simulink model "Track_model_wtihtesting_datacooling"  (R2024a)
settings: Solver=FixedStepAuto  StartTime=0.0  StopTime=1200  FixedStep=0.01  MaxStep=1e-2  MinStep=1e-5  RelTol=1e-3  AbsTol=1e-11
PreLoadFcn:
  | Straight1_Track = [75	3.446	29.063	1.834	47.653	8.247	3.373	13.154	57.193	39.54	5.916	3.204	2.701	2.747	90.673	4.72	3.366	94.658	23.788	1	40.161	15.969	17.891	3.717	36.358	76.419	54.208	36.993	4.775	55.007	1.783	4.349
  | ];
  | Curved_Track = [13.325	13.688	13.825	14.949	16.182	52.505	18.752	19.67	17.192	18.934	14.945	16.948	14.677	9.353	16.047	6.011	19.463	14.821	17.716	9.886	20.496	17.101	19.463	24.351	37.401	18.473	21.711	5.558	59.024	6.989	13.452	41.008
  | ];
  | Radius1 = [12	16.8	16.75	13.5	18.6	22.46	17.818	17.73	14	25.6	16.44	15.538	14.4	26.75	44.307	40	20.44	27.09	18.18	23.42	22.933	36.75	14.631	39	27.714	18.667	15.778	21.2	22.927	27.67	24.4	27.778
  | ];
model workspace (MAT data in the model file):
  Curve_Track = [19 13 16.3 21 23 16.5 21.6 28.81 24.6 43.9 54.836 13.8]
  Straight_Track = [35.7 53.5 32.527 50 30 20 11.2 36.6 21.4 41 38.7 74.5]
  Trac_vel = [10 5 8 12 8 9 10 9 11 14 10 10]
(part 2 of 2)

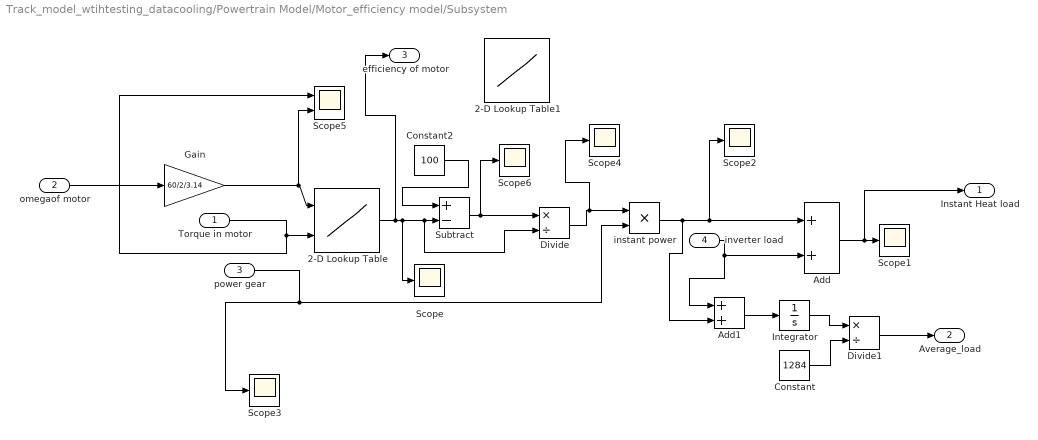
== system Track_model_wtihtesting_datacooling/Powertrain Model/Motor_efficiency model/Subsystem ==
  Torque in motor : Inport
  omegaof motor : Inport  Port=2
  power gear : Inport  Port=3
  inverter load : Inport  Port=4
  2-D Lookup Table : Lookup_n-D  BreakpointsForDimension1=[400;500;600;700;800;900;1000;1100;1200;1300;1400;1500;1600;1700;1800;1900;2000;2100;2200;2300;2400;2500;2600;2700;2800;2900;3000;3100;3200;3300;3400;3500;3600;3700;3800;3900;4000;4100;4200;4300;4400;4500;4600;4700;4800;4900;5000;5100;5200;5300;5400;5500;5600;5700;5800;5900;6000;6100;6200;6300;6400;6500;6600;6700;6800;6900;7000;7100;7200;7300;7400;7500;7600;7700;7800;7900;8000]  BreakpointsForDimension2=[6.9;8.9;10.9;12.9;14.9;16.9;18.9;20.9;22.9;24.9;26.9;28.9;30.9;32.9;34.9;36.9;38.9;40.9;42.9;44.9;46.9;48.9;50.9;52.9;54.9;56.9;58.9;60.9;62.9;64.9;66.9;68.9;70.9;72.9;74.9;76.9;78.9;80.9;82.9;84.9;86.9;88.9;90.9;92.9;94.9;96.9]  Table=[88 88.27289231 88.18254 88.21243 88.08233 88.08233 88.28824 88.28824 88.28824 88.28824 88.28824 88.28824 88.28824 88.28824 88.28824 88.28824 88.28824 88.28824 88.28824 88.28824 88.1819 87.5 87.65 88.5336 88.37676 88.1768 88 88.49353 88.23826 88 88.47392 88.19242 88 88.35438 88.05735 88.456 88.15094 88.48114 88.13851 88.39834 88 88.16702 88.28393 88.2702 88.05845 88;88 88.27289231 88.18254 88.21243 88.08233 88.08233 88.08233 88.25426 88.35324 88.41928 88.475 88.48092 88.47115 88.5 88.51281 88.46591 88.47674 88.39286 88.33757 88.28824 88.1819 88.05086 88 88.5336 88.37676 88.1768 88 88.49353 88.23826 88 88.47392 88.19242 88 88.35438 88.05735 88.456 88.15094 88.48114 88.13851 88.39834 88 88.16702 88.28393 88.2702 88.05845 88;88 88.27289231 88.18254 88.21243 88.21243 88.21243 88.49878 88.693 88.83121 88.93297 89.02333 89.08349 89.10385 89.17143 89.22128 89.20875 89.24186 89.17619 89.1209 89.09068 88.98434 88.84844 88.71707 88.5336 88.37676 88.1768 88 88.49353 88.23826 88 88.47392 88.19242 88 88.35438 88.05735 88.456 88.15094 88.48114 88.13851 88.39834 88 88.16702 88.28393 88.2702 88.05845 88;88 88.27289231 88.18254 88.18254 88.18254 88.56243 88.89114 89.12689 89.30917 89.43333 89.57167 89.68393 89.73654 89.84286 89.92128 89.93986 89.99049 89.95952 89.90976 89.89312 89.78678 89.64601 89.51951 89.32439 89.15482 88.94639 88.72378 88.49353 88.23826 88 88.47392 88.19242 88 88.35438 88.05735 88.456 88.15094 88.48114 88.13851 88.39834 88 88.16702 88.28393 88.2702 88.05845 88;88 88.27289231 88.01154 88.01154 88.48237 88.91132 89.26817 89.54334 89.77825 89.92267 90.10463 90.24673 90.36923 90.49795 90.6131 90.67097 90.73822 90.74286 90.7122 90.69556 90.58922 90.44359 90.30989 90.1209 89.92278 89.71598 89.48833 89.24696 88.99169 88.73085 88.47392 88.19242 88 88.35438 88.05735 88.456 88.15094 88.48114 88.13851 88.39834 88 88.16702 88.28393 88.2702 88.05845 88;88 88.27289231 88.27289 88.27289 88.77126 89.23138 89.61817 89.95213 90.17428 90.36607 90.59325 90.80877 90.96259 91.14729 91.29496 91.40208 91.48595 91.52619 91.51463 91.498 91.39166 91.24116 91.09792 90.90424 90.69689 90.48557 90.25344 90.0004 89.74513 89.47858 89.20475 88.92755 88.64335 88.35438 88.05735 88.456 88.15094 88.48114 88.13851 88.39834 88 88.16702 88.28393 88.2702 88.05845 88;88 88 88 88.52851 89.04043 89.52306 89.96107 90.31799 90.60371 90.8209 91.10465 91.3582 91.56326 91.79663 91.97683 92.00295 92.05952 92.10193 92.10227 92.05814 92.01129 92 91.88594 91.68757 91.47101 91.25296 91.0091 90.75383 90.49856 90.2263 89.92806 89.66412 89.37446 89.05438 88.76742 88.456 88.15094 88.48114 88.13851 88.39834 88 88.16702 88.28393 88.2702 88.05845 88;88 88.14920732 88.14921 88.73943 89.31372 89.80797 90.26084 90.67391 91.00435 91.302 91.5888 91.87495 92.03132 92.19548 92.31772 92.40417 92.45119 92.47579 92.47614 92.4407 92.39564 92.33926 92.25778 92.16175 92.04439 92 91.76253 91.50727 91.24569 90.97403 90.67017 90.38904 90.08981 89.77235 89.46813 89.13435 88.82237 88.48114 88.13851 88.39834 88 88.16702 88.28393 88.2702 88.05845 88;88 87.65 88.32909 88.95988 89.52772 90.08896 90.57269 91.00744 91.37299 91.71079 92 92.26103 92.4947 92.65 92.73951 92.80539 92.84286 92.84965 92.85 92.82326 92.77998 92.73093 92.659 92.5782 92.47166 92.35078 92.21438 92.04901 91.9768 91.69749 91.41227 91.10426 90.79733 90.47065 90.17443 89.82135 89.4938 89.15257 88.80315 88.39834 88 88.16702 88.28393 88.2702 88.05845 88;88 87.88 88.48154 89.13812 89.77055 90.316 90.85449 91.32356 91.72966 92.00037 92.39822 92.73588 92.97573 93.10637 93.16131 93.20661 93.23452 93.22352 93.22386 93.20581 93.16433 93.1226 93.06022 92.99466 92.89894 92.79538 92.66436 92.50865 92.35239 92.17744 92 91.81948 91.51013 91.16328 90.85062 90.50645 90.16522 89.80558 89.44756 89.05992 88.63094 88.16702 88.28393 88.2702 88.05845 88;88 88 88.63262 89.29166 89.95641 90.58122 91.10428 91.62176 92 92.43326 92.86929 93.21521 93.46267 93.55912 93.58684 93.60783 93.62619 93.59738 93.59773 93.58837 93.54867 93.51951 93.46144 93.41111 93.32621 ...(+22768 chars)]  InternalRulePriority=Speed  RndMeth=Simplest
      settings: InputPortMap=u0,u1
  2-D Lookup Table1 : Lookup_n-D  BreakpointsForDimension1=[0;500;1000;1500;1700;1800;1900;2000;2100;2300;2500;2600;2800;3000;3200;3400;3600;3800;4000;4200;4400;4600;4800;5000;5200;5400;5600;5800;6000;7000;8000]  BreakpointsForDimension2=[0;5;10;15;20;22;24;25;26;28;30;31;32;34;35;37;39;40;42;44;46;48;50;52;54;56;58;60;70;80;90]  Table=[82 82 82 82 82 82 82 82 82 82 82 82 82 82 82 82 82 82 82 82 82 82 82 82 82 82 82 82 82 82 82;82 82 82 82 86 86 86 86 86 86 86 86 86 86 86 86 86 86 86 86 86 86 86 86 82 82 82 82 82 82 82;82 82 82 86 86 86 86 86 86 86 86 86 86 90 90 90 90 90 90 90 90 90 90 86 86 86 86 86 86 86 82;82 82 86 86 86 90 90 90 90 90 90 90 94 94 94 94 94 94 94 94 90 90 90 90 90 90 90 90 90 86 86;82 82 86 86 90 90 90 90 90 94 94 94 94 94 94 94 94 94 94 94 94 94 94 94 94 94 94 94 90 90 86;82 82 86 86 90 90 90 90 90 94 94 94 94 94 94 94 94 94 94 94 94 94 94 94 94 94 94 94 90 90 86;82 82 86 86 90 90 90 90 90 94 94 94 94 94 94 94 94 94 94 94 94 94 94 94 95 95 95 95 94 90 86;82 82 86 86 90 90 90 94 94 94 94 94 94 94 94 94 94 94 94 94 94 94 95 95 95 95 95 95 94 90 86;82 82 86 86 90 90 90 94 94 94 94 94 94 94 94 94 94 94 94 94 95 95 95 95 95 95 95 95 94 90 86;82 82 86 86 90 90 90 94 94 94 94 94 94 94 94 94 95 95 95 95 95 95 95 95 95 95 95 95 94 90 86;82 82 86 86 90 90 90 94 94 94 94 94 94 94 94 95 95 95 95 95 96 96 96 96 96 96 95 95 94 90 86;82 82 86 86 90 90 90 94 94 94 94 94 94 95 95 95 95 95 95 96 96 96 96 96 96 96 95 95 94 90 86;82 82 86 86 90 90 94 94 94 94 95 95 95 95 96 96 96 96 96 96 96 96 96 96 96 96 95 95 94 90 86;82 82 86 86 90 90 94 94 94 94 95 95 95 95 96 96 96 96 96 96 96 96 96 96 96 96 95 95 94 90 86;82 82 86 86 90 90 94 94 94 95 95 95 96 96 96 96 96 96 96 96 96 96 96 96 96 96 95 95 94 94 86;82 82 86 86 90 90 94 94 94 95 95 95 96 96 96 96 96 96 96 96 96 96 96 96 96 96 95 95 94 94 86;82 82 86 86 90 90 90 94 94 95 95 95 96 96 96 96 96 96 96 96 96 96 96 96 96 96 95 95 94 94 86;82 82 86 86 90 90 94 94 94 95 95 95 96 96 96 96 96 96 96 96 96 96 96 96 96 95 95 95 94 94 86;82 82 86 86 90 90 94 94 94 95 95 95 95 96 96 96 96 96 96 96 96 96 96 96 96 95 95 95 94 94 86;82 82 86 86 90 90 94 94 94 95 95 95 95 96 96 96 96 96 96 96 96 96 96 96 96 95 95 95 94 94 86;82 82 86 86 90 90 94 94 94 94 95 95 95 95 96 96 96 96 96 96 96 96 96 96 96 95 95 95 94 94 86;82 82 86 86 90 90 94 94 94 94 95 95 95 95 96 96 96 96 96 96 96 96 96 96 96 95 95 95 94 94 86;82 82 86 86 90 90 94 94 94 94 94 94 95 95 95 96 96 96 96 96 96 96 96 96 96 95 95 95 94 94 86;82 82 86 86 90 90 94 94 94 94 94 94 95 95 95 96 96 96 96 96 96 96 96 96 95 95 95 95 94 94 86;82 82 86 86 90 90 94 94 94 94 94 94 94 95 95 95 96 96 96 96 96 96 96 96 95 95 95 95 94 94 86;82 82 86 86 90 90 94 90 94 94 94 94 94 94 95 95 95 96 96 96 96 96 96 96 95 95 95 95 94 94 86;82 82 86 86 90 90 90 90 94 94 94 94 94 94 95 95 95 95 95 95 95 95 95 95 95 95 95 95 94 94 86;82 82 86 82 90 90 90 90 94 94 94 94 94 94 94 94 95 95 95 95 95 95 95 95 95 95 95 95 94 94 86;82 82 82 82 90 90 90 90 94 94 94 94 94 94 94 94 95 95 95 95 95 95 95 95 95 95 95 95 94 94 86;82 82 82 82 86 86 86 86 86 86 90 90 90 90 90 90 94 94 94 94 94 94 94 94 94 94 94 94 94 90 86;82 82 82 82 82 82 82 82 82 82 82 82 82 82 82 82 82 82 82 86 86 86 86 90 90 90 90 90 94 94 82]  InternalRulePriority=Speed  RndMeth=Simplest
      settings: InputPortMap=u0,u1
  Add : Sum
  Add1 : Sum
  Constant : Constant  Value=1284
  Constant2 : Constant  Value=100
  Divide : Product  Inputs=*/
  Divide1 : Product  Inputs=*/
  Gain : Gain  Gain=60/2/3.14
  Integrator : Integrator
  Scope{,1..4,6} (6 alike) : Scope
  Scope5 : Scope  NumInputPorts=2
  Subtract : Sum  Inputs=+-
  instant power : Product  Inputs=**
  Instant Heat load : Outport
  Average_load : Outport  Port=2
  efficiency of motor : Outport  Port=3
  wires:
  power gear/1 -> instant power/2, Scope3/1
  Constant2/1 -> Subtract/1
  2-D Lookup Table/1 -> efficiency of motor/1, Scope/1, Divide/2, Subtract/2
  Subtract/1 -> Scope6/1, Divide/1
  Integrator/1 -> Divide1/1
  Divide/1 -> Scope4/1, instant power/1
  Constant/1 -> Divide1/2
  Divide1/1 -> Average_load/1
  Torque in motor/1 -> Scope5/1, 2-D Lookup Table/2
  omegaof motor/1 -> Gain/1
  Gain/1 -> Scope5/2, 2-D Lookup Table/1
  Add/1 -> Instant Heat load/1, Scope1/1
  inverter load/1 -> Add1/1, Add/2
  instant power/1 -> Scope2/1, Add/1, Add1/2
  Add1/1 -> Integrator/1

== matlab function Track_model_wtihtesting_datacooling/Powertrain Model/MATLAB Function1 ==
  data: u input; y output; data input
function y = fcn(u, data)
if u >=200
    y = 1;
else
    y = 0;
end

== matlab function Track_model_wtihtesting_datacooling/Deceleration of car/Frictional Force Evaluator/Friction Co-efficients ==
  data: Nf input; uF output; Nr input; uR output
function [uF , uR] = fcn(Nf , Nr)
safety_factor = 0.66;
uF = 2.9 - (0.14/300)*(Nf-600);
uR = 2.9 - (0.14/300)*(Nr-600);
uF = safety_factor*uF;
uR = safety_factor*uR;

== matlab function Track_model_wtihtesting_datacooling/Run Condition check/MATLAB Function ==
  data: distance input; effec_acc output; velocity input; acce input; dec input; straight input; curve input; traction_velocity input; Max_car_speed input; i input; cover_length input; i output; cover_length output; stop_condn output
function [effec_acc,i,cover_length,stop_condn] = fcn(distance,velocity,acce,dec,straight,curve,traction_velocity,Max_car_speed, i,cover_length)
stop_condn = 0;
if distance>22000
    stop_condn = 1;
end
    if  (i==0)
        i=+1;
    end
    if i>32
        i = 1; 
    end
   
    checklength = cover_length + straight(i);
       if distance<= (checklength - (traction_velocity(i)^2 - velocity^2)/(2*dec))  && (distance<= checklength)
         if velocity>Max_car_speed
             effec_acc = 0;
         else
           effec_acc = acce;
         end
       elseif (distance>= (checklength - (traction_velocity(i)^2 - velocity^2)/(2*dec))) && (distance<= checklength)
           effec_acc = dec;
       elseif (distance<= (checklength - (traction_velocity(i)^2 - velocity^2)/(2*dec))) && (distance>= checklength)
           effec_acc = 0;
       elseif (distance>= checklength) && (distance<= checklength +curve(i))
           effec_acc = 0;
       else
           cover_length = checklength + curve(i);
           effec_acc = acce;
           i= i+1;
       end
end

== matlab function Track_model_wtihtesting_datacooling/Deceleration of car/Weight Distribution ==
  data: wheelBase input; wF output; cgFromFrontAxle input; wR output
function [wF,wR ] = fcn(wheelBase , cgFromFrontAxle)
wR = cgFromFrontAxle / wheelBase;
wF = 1-wR;

== matlab function Track_model_wtihtesting_datacooling/Lateral Dynamics model/Lateral load transfer/LATERAL LOAD TRANSFER ==
  data: K_Arb input; mass input; lateral_acc input; N_F_inner output; unused input; N_F_outer output; N_R_inner output; N_R_outer output; roll output
function [N_F_inner,N_F_outer,N_R_inner,N_R_outer,roll] = fcn(K_Arb,mass,lateral_acc,~)

rc_h_f=0.05;
rc_h_r=0.07;
h_cg=0.235;
g=9.81;
m_f=0.46*mass;
m_r=0.54*mass;
k_s_front=302;
k_s_rear=300;
tw_f=1.250;
tw_r=1.2;
k_t_front=k_s_front+K_Arb(1);
k_t_rear =k_s_rear+K_Arb(2);
roll=(m_f*(h_cg-rc_h_f)+m_r*(h_cg-rc_h_r))*lateral_acc^2/((k_t_rear+k_t_front)*g);
force_transfer_front=m_f*rc_h_f*lateral_acc/tw_f+k_t_front*(m_f*(h_cg-rc_h_f)+m_r*(h_cg-rc_h_r))*lateral_acc/(tw_f*(k_t_rear+k_t_front));
force_transfer_rear=m_r*rc_h_r*lateral_acc/tw_r+k_t_rear*(m_f*(h_cg-rc_h_f)+m_r*(h_cg-rc_h_r))*lateral_acc/(tw_r*(k_t_rear+k_t_front));
N_F_inner=m_f*g/2-force_transfer_front;
N_F_outer=m_f*g/2+force_transfer_front;
N_R_inner=m_r*g/2-force_transfer_rear;
N_R_outer=m_r*g/2+force_transfer_rear;
end

== matlab function Track_model_wtihtesting_datacooling/Powertrain Model/Power Required at wheel/MATLAB Function ==
  data: Torque_ input; cir_tor input; constant_tor input; effec_accele input; effec_Tor output
function effec_Tor = fcn(Torque_, cir_tor, constant_tor, effec_accele)
if effec_accele>0
    effec_Tor = Torque_;
elseif effec_accele == 0
    effec_Tor = constant_tor;
else
    effec_Tor =0;
end

== matlab function Track_model_wtihtesting_datacooling/Powertrain Model/Accumulator Model/MATLAB Function ==
  data: OCV input; Resistance input; Term_vol output; current input
function Term_vol = fcn(OCV,Resistance,current)
Term_vol = OCV - current*Resistance;
end

== matlab function Track_model_wtihtesting_datacooling/Powertrain Model/Power_electronics/MATLAB Function ==
  data: Vdc input; Base_speed output; Idc input
function Base_speed  = fcn(Vdc,Idc)
Ld = 92e-6;     %Internal  Parameter of motor(d -axis inductance)
Lq = 102e-6;     %Internal  Parameter of motor(q -axis inductance)

L_dq = Ld- (Lq);    %intermediate calculation step
psi_f = 0.0299;     %
P=20;       %No of poles
K_t= 3*P/4;     %What is K_t?

V_r = Vdc/2;
y = 9*(V_r*psi_f)^2 - 4* (0.95*Vdc*Idc*Lq)^2;  %intermediate cal step in current circle eqn
m = (4 * (0.95*Vdc*Idc*psi_f)^2)/(y);   %modulation index we took safey factor of more than 10%, assuming that initally space-vector modulation was used.
iq = (m) %id is q-axis current
id=0; %id is d-axis current
wb = (V_r)/((Ld*id + psi_f)^2 + (Lq* iq)^2); %Electrical speed(speed in electrical domain)
Base_speed = wb*30*2/(pi*P) %Mechanical rpm of motor
end

== matlab function Track_model_wtihtesting_datacooling/Powertrain Model/VCU code ==
  data: Current input; Power_wheel input; Omega input; Set_Torque input; previous_power input; con_power output; Torque output
function [con_power,Torque]  = fcn(Current, Power_wheel,Omega, Set_Torque, previous_power)
if Current ==200
   con_power = Power_wheel;
   Torque = Power_wheel/Omega;
elseif Current >=200 && Current <=205
    con_power = previous_power;
    Torque = previous_power/Omega;
elseif Current >=205
    con_power = 31000;
    Torque = con_power/Omega;
else
    con_power =Power_wheel;
    Torque = Set_Torque;
end
